simulink model "blackbox_simulink_controller"  (R2016a)
settings: Solver=VariableStepAuto  StartTime=0.0  StopTime=10.0  RelTol=1e-3
undefined symbols (not defined in the file): OE_ss_CW
libraries: simulink x1
settings Model: Creator=Dick  LastModifiedBy=Dick

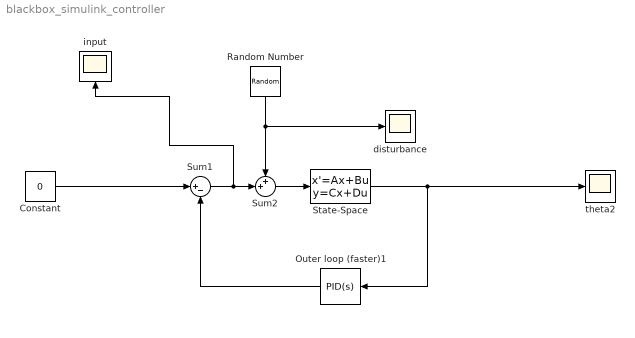
== system blackbox_simulink_controller ==
  Constant : Constant  Value=0
  Outer loop (faster)1 : simulink/Continuous/PID Controller  Controller=PID  TimeDomain=Continuous-time  SampleTime=-1  IntegratorMethod=Forward Euler  FilterMethod=Forward Euler  Form=Parallel  UseFilter=on  ControllerParametersSource=internal  P=10  I=3  D=0  N=100  InitialConditionSource=internal  InitialConditionForIntegrator=0  InitialConditionForFilter=0  ExternalReset=none  LimitOutput=off  UpperSaturationLimit=inf  LowerSaturationLimit=-inf  LinearizeAsGain=on  AntiWindupMode=none  Kb=1  TrackingMode=off  Kt=1  PParamMin=[]  PParamMax=[]  IParamMin=[]  IParamMax=[]  DParamMin=[]  DParamMax=[]  NParamMin=[]  NParamMax=[]  KbParamMin=[]  KbParamMax=[]  KtParamMin=[]  KtParamMax=[]  POutMin=[]  POutMax=[]  IOutMin=[]  IOutMax=[]  DOutMin=[]  DOutMax=[]  NOutMin=[]  NOutMax=[]  KbOutMin=[]  KbOutMax=[]  KtOutMin=[]  KtOutMax=[]  IntegratorOutMin=[]  IntegratorOutMax=[]  FilterOutMin=[]  FilterOutMax=[]  SumOutMin=[]  SumOutMax=[]  SumI1OutMin=[]  SumI1OutMax=[]  SumI2OutMin=[]  SumI2OutMax=[]  SumI3OutMin=[]  SumI3OutMax=[]  SumDOutMin=[]  SumDOutMax=[]  SaturationOutMin=[]  SaturationOutMax=[]  IntegratorContinuousStateAttributes=''  IntegratorStateMustResolveToSignalObject=off  IntegratorRTWStateStorageClass=Auto  FilterContinuousStateAttributes=''  FilterStateMustResolveToSignalObject=off  FilterRTWStateStorageClass=Auto  DifferentiatorICPrevScaledInput=0  DifferentiatorOutMin=[]  DifferentiatorOutMax=[]
  Random Number : RandomNumber  Variance=0.5  SampleTime=5
  State-Space : StateSpace  A=OE_ss_CW.A  B=OE_ss_CW.B  C=OE_ss_CW.C  D=OE_ss_CW.D  X0=0  ContinuousStateAttributes='black_box_states'
  Sum1 : Sum  Inputs=|+-
  Sum2 : Sum  Inputs=++|
  disturbance : Scope
  input : Scope
  theta2 : Scope
  wires:
  Sum2/1 -> State-Space/1
  Random Number/1 -> Sum2/1, disturbance/1
  Sum1/1 -> input/1, Sum2/2
  Constant/1 -> Sum1/1
  Outer loop (faster)1/1 -> Sum1/2
  State-Space/1 -> Outer loop (faster)1/1, theta2/1
